simulink subsystem "Bball_Ref_Inputs"  (R2026a)
settings: Solver=VariableStepAuto
undefined symbols (not defined in the file): SimPar
libraries: BezierLib x1
settings Model: Creator=macheson  LastModifiedBy=pkmas

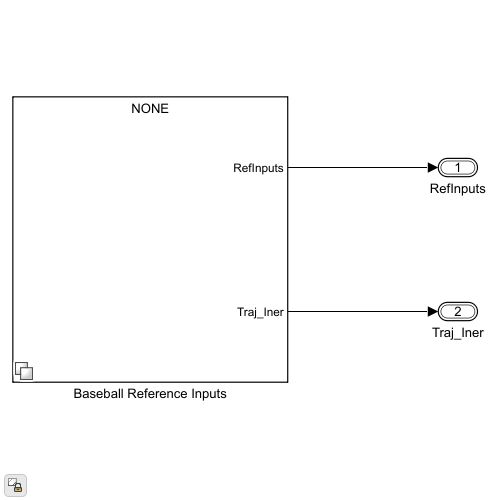
[thumbnail: Simulink's stored preview of the top-level diagram]
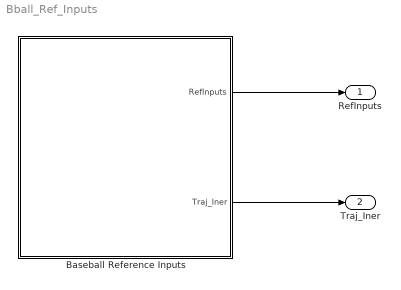
== system Bball_Ref_Inputs ==
  Baseball Reference Inputs : Subsystem  Variant=on
  RefInputs : Outport  OutDataTypeStr=Bus: BUS_REF_INPUT
  Traj_Iner : Outport  Port=2  OutDataTypeStr=Bus: BUS_REF_INPUT_INER
  wires:
  Baseball Reference Inputs/1(RefInputs) -> RefInputs/1
  Baseball Reference Inputs/2(Traj_Iner) -> Traj_Iner/1

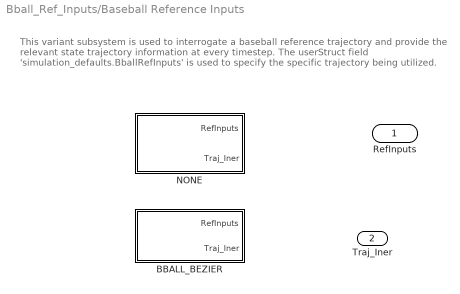
== system Bball_Ref_Inputs/Baseball Reference Inputs ==
  note: This variant subsystem is used to interrogate a baseball reference trajectory
      | and provide the relevant state trajectory information at every timestep. The userStruct field 'simulation_defaults.BballRefInputs' is used to specify the specific trajectory being utilized.
  BBALL_BEZIER : Subsystem  VariantControl=GVS_BBALL_REFINPUT_TYPE_BEZIER
  NONE : Subsystem  VariantControl=GVS_BBALL_REFINPUT_TYPE_NONE
  RefInputs : Outport  OutDataTypeStr=Bus: BUS_REF_INPUT
  Traj_Iner : Outport  Port=2  OutDataTypeStr=Bus: BUS_REF_INPUT_INER

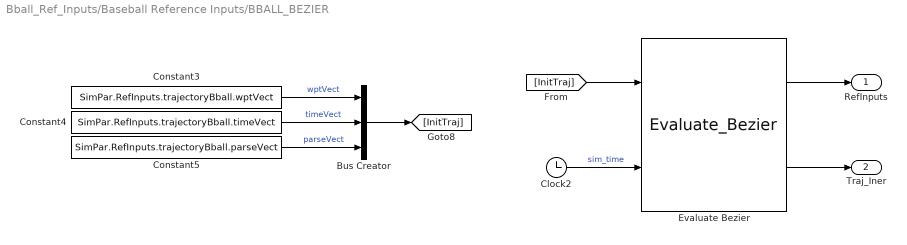
== system Bball_Ref_Inputs/Baseball Reference Inputs/BBALL_BEZIER ==
  Bus Creator : BusCreator  Inputs=3
  Clock2 : Clock
  Constant3 : Constant  Value=SimPar.RefInputs.trajectoryBball.wptVect
  Constant4 : Constant  Value=SimPar.RefInputs.trajectoryBball.timeVect
  Constant5 : Constant  Value=SimPar.RefInputs.trajectoryBball.parseVect
  Evaluate Bezier : BezierLib/Evaluate_Bezier  tlen_max=1
  RefInputs : Outport
  Traj_Iner : Outport  Port=2
  wires:
  Constant4/1 -> Bus Creator/2  "timeVect"
  Evaluate Bezier/2 -> Traj_Iner/1
  Constant5/1 -> Bus Creator/3  "parseVect"
  [InitTraj] -> Evaluate Bezier/1
  Clock2/1 -> Evaluate Bezier/2  "sim_time"
  Constant3/1 -> Bus Creator/1  "wptVect"
  Evaluate Bezier/1 -> RefInputs/1
  Bus Creator/1 -> [InitTraj]

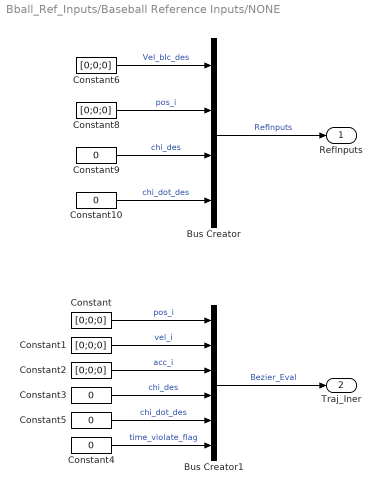
== system Bball_Ref_Inputs/Baseball Reference Inputs/NONE ==
  Bus Creator : BusCreator  Inputs=4
  Bus Creator1 : BusCreator  Inputs=6
  Constant{,1..2,6,8} (5 alike) : Constant  Value=[0;0;0]
  Constant{3..5,9..10} (5 alike) : Constant  Value=0
  RefInputs : Outport
  Traj_Iner : Outport  Port=2
  wires:
  Constant2/1 -> Bus Creator1/3  "acc_i"
  Constant5/1 -> Bus Creator1/5  "chi_dot_des"
  Constant10/1 -> Bus Creator/4  "chi_dot_des"
  Constant4/1 -> Bus Creator1/6  "time_violate_flag"
  Bus Creator/1 -> RefInputs/1  "RefInputs"
  Constant9/1 -> Bus Creator/3  "chi_des"
  Constant/1 -> Bus Creator1/1  "pos_i"
  Constant6/1 -> Bus Creator/1  "Vel_bIc_des"
  Bus Creator1/1 -> Traj_Iner/1  "Bezier_Eval"
  Constant8/1 -> Bus Creator/2  "pos_i"
  Constant1/1 -> Bus Creator1/2  "vel_i"
  Constant3/1 -> Bus Creator1/4  "chi_des"
